simulink library "Control_Library_Rev2"  (R2020b)
settings: Solver=VariableStepAuto  StartTime=0.0  StopTime=10.0  RelTol=1e-3
values from neighbouring files (symbols this model uses):
  Controller_sampleTime = 0.001    [PLC_setup_Rev1_02Mar21.m]    (also in PLC_setup_Rev3.m; PLC_setup_Rev4.m)
  Droop_scaling = 0    [PLC_setup_Rev1_02Mar21.m]    (also in PLC_setup_Rev3.m; PLC_setup_Rev4.m)
  VFD_Adapt_factor_lower_p1458 = 1    [PLC_setup_Rev1_02Mar21.m]    (also in PLC_setup_Rev3.m; PLC_setup_Rev4.m)
  VFD_Adapt_factor_upper_p1459 = 1    [PLC_setup_Rev1_02Mar21.m]    (also in PLC_setup_Rev3.m; PLC_setup_Rev4.m)
  VFD_Curr_limit_var_p0641 = 1    [PLC_setup_Rev1_02Mar21.m]    (also in PLC_setup_Rev3.m; PLC_setup_Rev4.m)
  VFD_Current_limit_p0640 = 430    [PLC_setup_Rev1_02Mar21.m]    (also in PLC_setup_Rev3.m; PLC_setup_Rev4.m)
  VFD_Id_setp_total_r1624 = 73    [PLC_setup_Rev1_02Mar21.m]    (also in PLC_setup_Rev3.m; PLC_setup_Rev4.m)
  VFD_Iq = 1    [PLC_setup_Rev1_02Mar21.m]    (also in PLC_setup_Rev3.m; PLC_setup_Rev4.m)
  VFD_Kp_n_basic_p1460 = 20.174    [PLC_setup_Rev1_02Mar21.m]    (also in PLC_setup_Rev3.m; PLC_setup_Rev4.m)
  VFD_M = inf    [PLC_setup_Rev1_02Mar21.m]    (also in PLC_setup_Rev3.m; PLC_setup_Rev4.m)
  VFD_M_accel_T_smooth_p1517 = 4    [PLC_setup_Rev1_02Mar21.m]    (also in PLC_setup_Rev3.m; PLC_setup_Rev4.m)
  VFD_M_lim_var_fixS_src_p1551 = 1    [PLC_setup_Rev1_02Mar21.m]    (also in PLC_setup_Rev3.m; PLC_setup_Rev4.m)
  VFD_M_max_lower_p1521 = -1345    [PLC_setup_Rev1_02Mar21.m]    (also in PLC_setup_Rev3.m; PLC_setup_Rev4.m)
  VFD_M_max_lower_scal_p1525 = 1    [PLC_setup_Rev1_02Mar21.m]    (also in PLC_setup_Rev3.m; PLC_setup_Rev4.m)
  VFD_M_max_up_mot_scal_p1524 = 1    [PLC_setup_Rev1_02Mar21.m]    (also in PLC_setup_Rev3.m; PLC_setup_Rev4.m)
  VFD_M_max_upper_p1520 = 1345    [PLC_setup_Rev1_02Mar21.m]    (also in PLC_setup_Rev3.m; PLC_setup_Rev4.m)
  VFD_n_act_T_smooth_p1442 = 4    [PLC_setup_Rev1_02Mar21.m]    (also in PLC_setup_Rev3.m; PLC_setup_Rev4.m)
  VFD_n_ctr_Kp_n_up_scal_p1461 = 1    [PLC_setup_Rev1_02Mar21.m]    (also in PLC_setup_Rev3.m; PLC_setup_Rev4.m)
  VFD_n_ctr_Tn_n_up_sca_p1463 = 1    [PLC_setup_Rev1_02Mar21.m]    (also in PLC_setup_Rev3.m; PLC_setup_Rev4.m)
  VFD_n_ctrl_adapt_Kp_lower_p1456 = 0    [PLC_setup_Rev1_02Mar21.m]    (also in PLC_setup_Rev3.m; PLC_setup_Rev4.m)
  VFD_n_ctrl_adapt_Kp_upper_p1457 = 0.1    [PLC_setup_Rev1_02Mar21.m]    (also in PLC_setup_Rev3.m; PLC_setup_Rev4.m)
  VFD_n_ctrl_Adpt_sig_Kp_p1455 = 0    [PLC_setup_Rev1_02Mar21.m]    (also in PLC_setup_Rev3.m; PLC_setup_Rev4.m)
  VFD_n_ctrl_Kp_scal_p1466 = 1    [PLC_setup_Rev1_02Mar21.m]    (also in PLC_setup_Rev3.m; PLC_setup_Rev4.m)
  VFD_n_ctrl_n_lower_p1464 = 0    [PLC_setup_Rev1_02Mar21.m]    (also in PLC_setup_Rev3.m; PLC_setup_Rev4.m)
  VFD_n_ctrl_n_upper_p1465 = 1680    [PLC_setup_Rev1_02Mar21.m]    (also in PLC_setup_Rev3.m; PLC_setup_Rev4.m)
  VFD_n_ctrl_Tn_n_lower_p1462 = 96    [PLC_setup_Rev1_02Mar21.m]    (also in PLC_setup_Rev3.m; PLC_setup_Rev4.m)
  VFD_n_limit_neg_p1086 = -40000    [PLC_setup_Rev1_02Mar21.m]    (also in PLC_setup_Rev3.m; PLC_setup_Rev4.m)
  VFD_n_limit_pos_p1083 = 40000    [PLC_setup_Rev1_02Mar21.m]    (also in PLC_setup_Rev3.m; PLC_setup_Rev4.m)
  VFD_n_limit_setp_p1063 = 40000    [PLC_setup_Rev1_02Mar21.m]    (also in PLC_setup_Rev3.m; PLC_setup_Rev4.m)
  VFD_n_max_p1082 = 1680    [PLC_setup_Rev1_02Mar21.m]    (also in PLC_setup_Rev3.m; PLC_setup_Rev4.m)
  VFD_n_set_filt_1_T_p1416 = 0    [PLC_setup_Rev1_02Mar21.m]    (also in PLC_setup_Rev3.m; PLC_setup_Rev4.m)
  VFD_P_max_gen_p1531 = -375    [PLC_setup_Rev1_02Mar21.m]    (also in PLC_setup_Rev3.m; PLC_setup_Rev4.m)
  VFD_P_max_mot_p1530 = 125    [PLC_setup_Rev1_02Mar21.m]    (also in PLC_setup_Rev3.m; PLC_setup_Rev4.m)
  VFD_PU_I_outp_max_r0289 = 452    [PLC_setup_Rev1_02Mar21.m]    (also in PLC_setup_Rev3.m; PLC_setup_Rev4.m)
  VFD_RFG_ramp_down_time_p1121 = 0.7    [PLC_setup_Rev1_02Mar21.m]    (also in PLC_setup_Rev3.m; PLC_setup_Rev4.m)
  VFD_RFG_ramp_up_time_p1120 = 0.7    [PLC_setup_Rev1_02Mar21.m]    (also in PLC_setup_Rev3.m; PLC_setup_Rev4.m)
  VFD_RFG_t_RD_scal_p1139 = 1    [PLC_setup_Rev1_02Mar21.m]    (also in PLC_setup_Rev3.m; PLC_setup_Rev4.m)
  VFD_RFG_t_RU_scal_p1138 = 1    [PLC_setup_Rev1_02Mar21.m]    (also in PLC_setup_Rev3.m; PLC_setup_Rev4.m)
undefined symbols (not defined in the file or in its folder): DiscIntNeverNeededParam
libraries: simulink x24, $bdroot x2
settings Model: Creator=JillMacPherson  LastModifiedBy=JillMacPherson

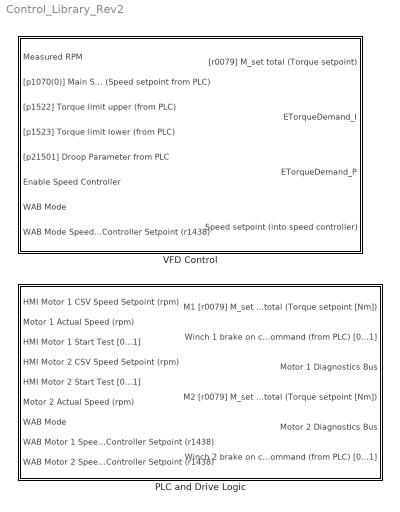
== system Control_Library_Rev2 ==
  PLC and Drive Logic : Subsystem
  VFD Control : Subsystem  TreatAsAtomicUnit=on  SystemSampleTime=Controller_sampleTime

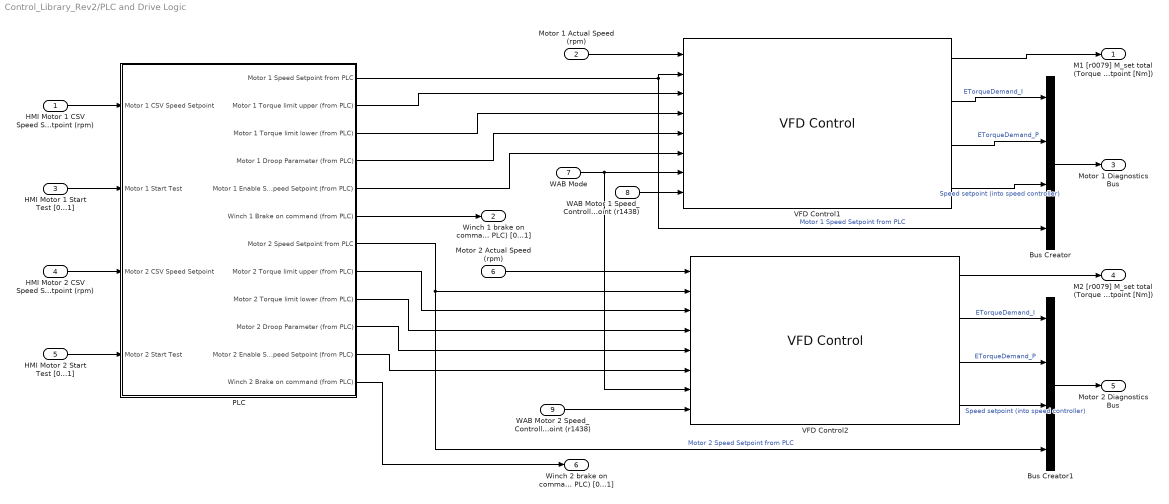
== system Control_Library_Rev2/PLC and Drive Logic ==
  HMI Motor 1 CSV Speed Setpoint (rpm) : Inport
  Motor 1 Actual Speed (rpm) : Inport  Port=2
  HMI Motor 1 Start Test [0...1] : Inport  Port=3
  HMI Motor 2 CSV Speed Setpoint (rpm) : Inport  Port=4
  HMI Motor 2 Start Test [0...1] : Inport  Port=5
  Motor 2 Actual Speed (rpm) : Inport  Port=6
  WAB Mode : Inport  Port=7
  WAB Motor 1 Speed_Controller Setpoint (r1438) : Inport  Port=8
  WAB Motor 2 Speed_Controller Setpoint (r1438) : Inport  Port=9
  Bus Creator : BusCreator  Inputs=4
  Bus Creator1 : BusCreator  Inputs=4
  PLC : Subsystem  TreatAsAtomicUnit=on  SystemSampleTime=Controller_sampleTime
  VFD Control1 : $bdroot/VFD Control  SystemSampleTime=Controller_sampleTime  VariantActivationTime=update diagram  Latency=0  AutoFrameSizeCalculation=off
  VFD Control2 : $bdroot/VFD Control  SystemSampleTime=Controller_sampleTime  VariantActivationTime=update diagram  Latency=0  AutoFrameSizeCalculation=off
  M1 [r0079] M_set total (Torque setpoint [Nm]) : Outport
  Winch 1 brake on command (from PLC) [0...1] : Outport  Port=2
  Motor 1 Diagnostics Bus : Outport  Port=3
  M2 [r0079] M_set total (Torque setpoint [Nm]) : Outport  Port=4
  Motor 2 Diagnostics Bus : Outport  Port=5
  Winch 2 brake on command (from PLC) [0...1] : Outport  Port=6
  wires:
  WAB Motor 2 Speed_Controller Setpoint (r1438)/1 -> VFD Control2/8
  WAB Mode/1 -> VFD Control1/7, VFD Control2/7
  WAB Motor 1 Speed_Controller Setpoint (r1438)/1 -> VFD Control1/8
  PLC/12(Winch 2 Brake on command (from PLC)) -> Winch 2 brake on command (from PLC) [0...1]/1
  PLC/11(Motor 2 Enable Speed Setpoint (from PLC)) -> VFD Control2/6
  PLC/10(Motor 2 Droop Parameter (from PLC)) -> VFD Control2/5
  PLC/9(Motor 2 Torque limit lower (from PLC)) -> VFD Control2/4
  PLC/8(Motor 2 Torque limit upper (from PLC)) -> VFD Control2/3
  PLC/7(Motor 2 Speed Setpoint from PLC) -> VFD Control2/2, Bus Creator1/4  "Motor 2 Speed Setpoint from PLC"
  Motor 2 Actual Speed (rpm)/1 -> VFD Control2/1
  HMI Motor 2 Start Test [0...1]/1 -> PLC/4(Motor 2 Start Test)
  HMI Motor 2 CSV Speed Setpoint (rpm)/1 -> PLC/3(Motor 2 CSV Speed Setpoint)
  PLC/6(Winch 1 Brake on command (from PLC)) -> Winch 1 brake on command (from PLC) [0...1]/1
  VFD Control2/1 -> M2 [r0079] M_set total (Torque setpoint [Nm])/1
  VFD Control2/2 -> Bus Creator1/1  "ETorqueDemand_I"
  VFD Control2/3 -> Bus Creator1/2  "ETorqueDemand_P"
  VFD Control2/4 -> Bus Creator1/3  "Speed setpoint (into speed controller)"
  Bus Creator1/1 -> Motor 2 Diagnostics Bus/1
  Bus Creator/1 -> Motor 1 Diagnostics Bus/1
  VFD Control1/4 -> Bus Creator/3  "Speed setpoint (into speed controller)"
  VFD Control1/3 -> Bus Creator/2  "ETorqueDemand_P"
  VFD Control1/2 -> Bus Creator/1  "ETorqueDemand_I"
  PLC/5(Motor 1 Enable Speed Setpoint (from PLC)) -> VFD Control1/6
  PLC/4(Motor 1 Droop Parameter (from PLC)) -> VFD Control1/5
  HMI Motor 1 CSV Speed Setpoint (rpm)/1 -> PLC/1(Motor 1 CSV Speed Setpoint)
  VFD Control1/1 -> M1 [r0079] M_set total (Torque setpoint [Nm])/1
  HMI Motor 1 Start Test [0...1]/1 -> PLC/2(Motor 1 Start Test)
  PLC/1(Motor 1 Speed Setpoint from PLC) -> Bus Creator/4, VFD Control1/2  "Motor 1 Speed Setpoint from PLC"
  PLC/2(Motor 1 Torque limit upper (from PLC)) -> VFD Control1/3
  Motor 1 Actual Speed (rpm)/1 -> VFD Control1/1
  PLC/3(Motor 1 Torque limit lower (from PLC)) -> VFD Control1/4

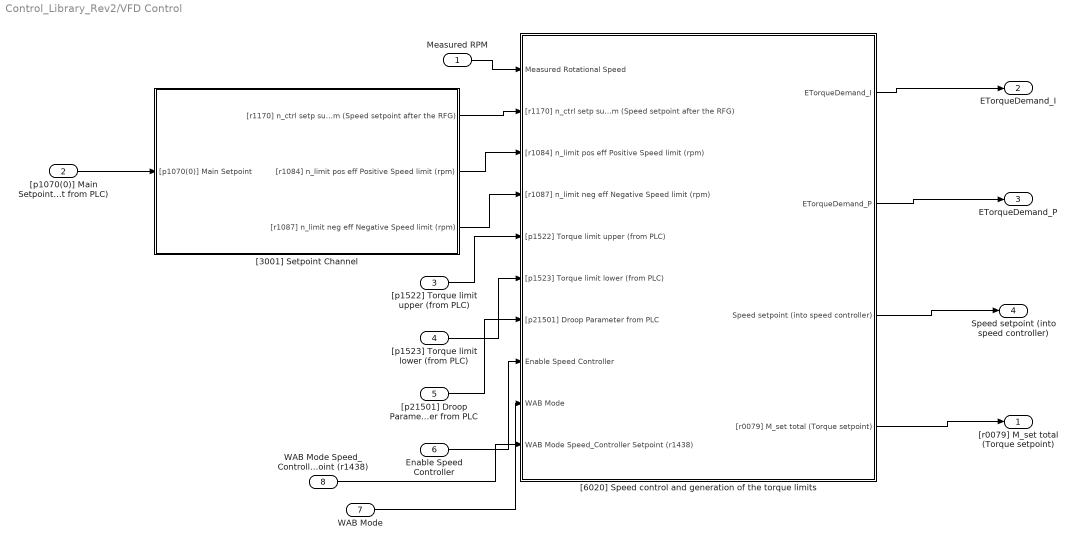
== system Control_Library_Rev2/VFD Control ==
  Measured RPM : Inport
  "[p1070(0)] Main Setpoint (Speed setpoint from PLC)" : Inport  Port=2
  "[p1522] Torque limit upper (from PLC)" : Inport  Port=3
  "[p1523] Torque limit lower (from PLC)" : Inport  Port=4
  "[p21501] Droop Parameter from PLC" : Inport  Port=5
  Enable Speed Controller : Inport  Port=6
  WAB Mode : Inport  Port=7
  WAB Mode Speed_Controller Setpoint (r1438) : Inport  Port=8
  "[3001] Setpoint Channel " : Subsystem
  "[6020] Speed control and generation of the torque limits " : Subsystem
  "[r0079] M_set total (Torque setpoint)" : Outport  VectorParamsAs1DForOutWhenUnconnected=off
  ETorqueDemand_I : Outport  Port=2  VectorParamsAs1DForOutWhenUnconnected=off
  ETorqueDemand_P : Outport  Port=3  VectorParamsAs1DForOutWhenUnconnected=off
  Speed setpoint (into speed controller) : Outport  Port=4  VectorParamsAs1DForOutWhenUnconnected=off
  wires:
  WAB Mode Speed_Controller Setpoint (r1438)/1 -> "[6020] Speed control and generation of the torque limits "/10(WAB Mode Speed_Controller Setpoint (r1438))
  WAB Mode/1 -> "[6020] Speed control and generation of the torque limits "/9(WAB Mode)
  "[6020] Speed control and generation of the torque limits "/1(ETorqueDemand_I) -> ETorqueDemand_I/1
  "[6020] Speed control and generation of the torque limits "/2(ETorqueDemand_P) -> ETorqueDemand_P/1
  Measured RPM/1 -> "[6020] Speed control and generation of the torque limits "/1(Measured Rotational Speed)
  "[p1070(0)] Main Setpoint (Speed setpoint from PLC)"/1 -> "[3001] Setpoint Channel "/1("[p1070(0)] Main Setpoint")
  "[3001] Setpoint Channel "/1("[r1170] n_ctrl setp sum (Speed setpoint after the RFG)") -> "[6020] Speed control and generation of the torque limits "/2("[r1170] n_ctrl setp sum (Speed setpoint after the RFG)")
  "[3001] Setpoint Channel "/2("[r1084] n_limit pos eff Positive Speed limit (rpm)") -> "[6020] Speed control and generation of the torque limits "/3("[r1084] n_limit pos eff Positive Speed limit (rpm)")
  "[3001] Setpoint Channel "/3("[r1087] n_limit neg eff Negative Speed limit (rpm)") -> "[6020] Speed control and generation of the torque limits "/4("[r1087] n_limit neg eff Negative Speed limit (rpm)")
  "[6020] Speed control and generation of the torque limits "/3(Speed setpoint (into speed controller)) -> Speed setpoint (into speed controller)/1
  "[6020] Speed control and generation of the torque limits "/4("[r0079] M_set total (Torque setpoint)") -> "[r0079] M_set total (Torque setpoint)"/1
  "[p1523] Torque limit lower (from PLC)"/1 -> "[6020] Speed control and generation of the torque limits "/6("[p1523] Torque limit lower (from PLC)")
  "[p1522] Torque limit upper (from PLC)"/1 -> "[6020] Speed control and generation of the torque limits "/5("[p1522] Torque limit upper (from PLC)")
  "[p21501] Droop Parameter from PLC"/1 -> "[6020] Speed control and generation of the torque limits "/7("[p21501] Droop Parameter from PLC")
  Enable Speed Controller/1 -> "[6020] Speed control and generation of the torque limits "/8(Enable Speed Controller)

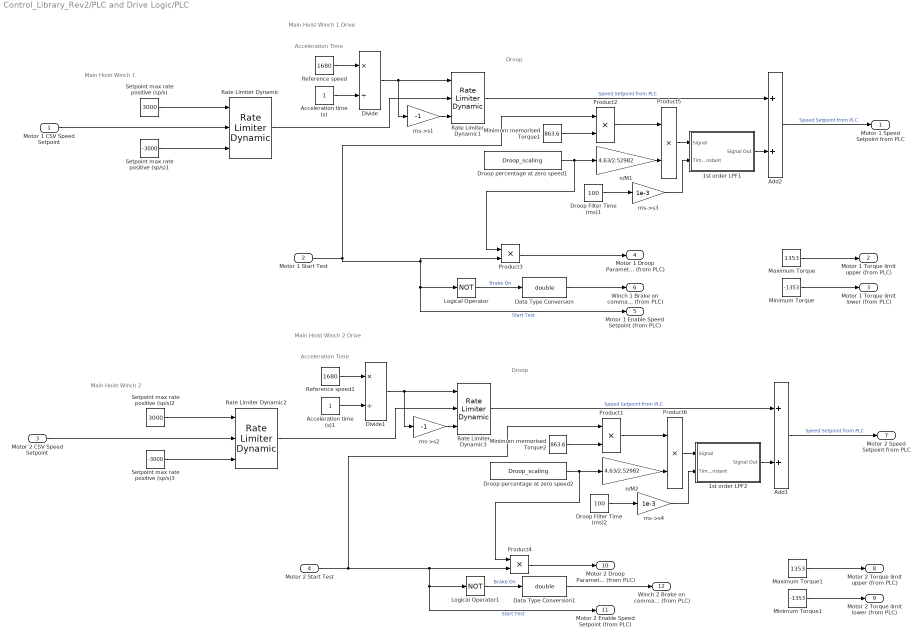
== system Control_Library_Rev2/PLC and Drive Logic/PLC ==
  note: Main Hoist Winch 2
  note: Droop
  note: Acceleration Time
  note: Main Hoist Winch 2 Drive
  note: Main Hoist Winch 1
  note: Droop
  note: Acceleration Time
  note: Main Hoist Winch 1 Drive
  Motor 1 CSV Speed Setpoint : Inport
  Motor 1 Start Test : Inport  Port=2
  Motor 2 CSV Speed Setpoint : Inport  Port=3
  Motor 2 Start Test : Inport  Port=4
  1st order LPF1 : Subsystem  mask{time_constant=0.1, Yo=0}
      mask prompts: time_constant "Time Constant (s)"; Yo "Initial Condition"
  1st order LPF2 : Subsystem  mask{time_constant=0.1, Yo=0}
      mask prompts: time_constant "Time Constant (s)"; Yo "Initial Condition"
  Acceleration time (s) : Constant
  Acceleration time (s)1 : Constant
  Add1 : Sum
  Add2 : Sum
  Data Type Conversion : DataTypeConversion  OutDataTypeStr=double
  Data Type Conversion1 : DataTypeConversion  OutDataTypeStr=double
  Divide : Product  Inputs=*/
  Divide1 : Product  Inputs=*/
  Droop Filter Time (ms)1 : Constant  Value=100
  Droop Filter Time (ms)2 : Constant  Value=100
  Droop percentage at zero speed1 : Constant  Value=Droop_scaling
  Droop percentage at zero speed2 : Constant  Value=Droop_scaling
  Logical Operator : Logic  Operator=NOT  AllPortsSameDT=off  OutDataTypeStr=boolean
  Logical Operator1 : Logic  Operator=NOT  AllPortsSameDT=off  OutDataTypeStr=boolean
  Maximum Torque : Constant  Value=1353
  Maximum Torque1 : Constant  Value=1353
  Minimum Torque : Constant  Value=-1353
  Minimum Torque1 : Constant  Value=-1353
  Minimum memorised Torque1 : Constant  Value=863.6
  Minimum memorised Torque2 : Constant  Value=863.6
  Product{1..2,5..6} (4 alike) : Product  Inputs=**
  Product3 : Product
  Product4 : Product
  Rate Limiter Dynamic{,1..3} (4 alike) : simulink/Discontinuities/Rate Limiter Dynamic
  Reference speed : Constant  Value=1680
  Reference speed1 : Constant  Value=1680
  Setpoint max rate positive (sp/s) : Constant  Value=3000
  Setpoint max rate positive (sp/s)1 : Constant  Value=-3000
  Setpoint max rate positive (sp/s)2 : Constant  Value=3000
  Setpoint max rate positive (sp/s)3 : Constant  Value=-3000
  ms->s1 : Gain  Gain=-1
  ms->s2 : Gain  Gain=-1
  ms->s3 : Gain  Gain=1e-3
  ms->s4 : Gain  Gain=1e-3
  n/M1 : Gain  Gain=4.63/2.52982
  n/M2 : Gain  Gain=4.63/2.52982
  Motor 1 Speed Setpoint from PLC : Outport
  Motor 1 Torque limit upper (from PLC) : Outport  Port=2
  Motor 1 Torque limit lower (from PLC) : Outport  Port=3
  Motor 1 Droop Parameter (from PLC) : Outport  Port=4
  Motor 1 Enable Speed Setpoint (from PLC) : Outport  Port=5
  Winch 1 Brake on command (from PLC) : Outport  Port=6
  Motor 2 Speed Setpoint from PLC : Outport  Port=7
  Motor 2 Torque limit upper (from PLC) : Outport  Port=8
  Motor 2 Torque limit lower (from PLC) : Outport  Port=9
  Motor 2 Droop Parameter (from PLC) : Outport  Port=10
  Motor 2 Enable Speed Setpoint (from PLC) : Outport  Port=11
  Winch 2 Brake on command (from PLC) : Outport  Port=12
  wires:
  Product1/1 -> Product6/1
  n/M2/1 -> Product6/2
  ms->s2/1 -> Rate Limiter Dynamic3/3
  ms->s4/1 -> 1st order LPF2/2(Time Constant)
  Divide1/1 -> ms->s2/1, Rate Limiter Dynamic3/1
  Setpoint max rate positive (sp/s)2/1 -> Rate Limiter Dynamic2/1
  Setpoint max rate positive (sp/s)3/1 -> Rate Limiter Dynamic2/3
  Product6/1 -> 1st order LPF2/1(Signal)
  Droop Filter Time (ms)2/1 -> ms->s4/1
  1st order LPF2/1(Signal Out) -> Add1/2
  Droop percentage at zero speed2/1 -> Product4/1, n/M2/1
  Rate Limiter Dynamic2/1 -> Rate Limiter Dynamic3/2
  Minimum memorised Torque2/1 -> Product1/2
  Reference speed1/1 -> Divide1/1
  Acceleration time (s)1/1 -> Divide1/2
  Add1/1 -> Motor 2 Speed Setpoint from PLC/1  "Speed Setpoint from PLC"
  Maximum Torque1/1 -> Motor 2 Torque limit upper (from PLC)/1
  Minimum Torque1/1 -> Motor 2 Torque limit lower (from PLC)/1
  Rate Limiter Dynamic3/1 -> Add1/1  "Speed Setpoint from PLC"
  Motor 2 Start Test/1 -> Product4/2, Logical Operator1/1, Motor 2 Enable Speed Setpoint (from PLC)/1, Product1/1  "Start Test"
  Product4/1 -> Motor 2 Droop Parameter (from PLC)/1
  Logical Operator1/1 -> Data Type Conversion1/1  "Brake On"
  Data Type Conversion1/1 -> Winch 2 Brake on command (from PLC)/1
  Motor 2 CSV Speed Setpoint/1 -> Rate Limiter Dynamic2/2
  Motor 1 CSV Speed Setpoint/1 -> Rate Limiter Dynamic/2
  Data Type Conversion/1 -> Winch 1 Brake on command (from PLC)/1
  Logical Operator/1 -> Data Type Conversion/1  "Brake On"
  Product3/1 -> Motor 1 Droop Parameter (from PLC)/1
  Motor 1 Start Test/1 -> Product2/1, Product3/2, Logical Operator/1, Motor 1 Enable Speed Setpoint (from PLC)/1  "Start Test"
  Rate Limiter Dynamic1/1 -> Add2/1  "Speed Setpoint from PLC"
  Minimum Torque/1 -> Motor 1 Torque limit lower (from PLC)/1
  Maximum Torque/1 -> Motor 1 Torque limit upper (from PLC)/1
  Add2/1 -> Motor 1 Speed Setpoint from PLC/1  "Speed Setpoint from PLC"
  Acceleration time (s)/1 -> Divide/2
  Reference speed/1 -> Divide/1
  Minimum memorised Torque1/1 -> Product2/2
  Rate Limiter Dynamic/1 -> Rate Limiter Dynamic1/2
  Droop percentage at zero speed1/1 -> n/M1/1, Product3/1
  1st order LPF1/1(Signal Out) -> Add2/2
  Droop Filter Time (ms)1/1 -> ms->s3/1
  Product5/1 -> 1st order LPF1/1(Signal)
  Setpoint max rate positive (sp/s)1/1 -> Rate Limiter Dynamic/3
  Setpoint max rate positive (sp/s)/1 -> Rate Limiter Dynamic/1
  Divide/1 -> Rate Limiter Dynamic1/1, ms->s1/1
  ms->s3/1 -> 1st order LPF1/2(Time Constant)
  ms->s1/1 -> Rate Limiter Dynamic1/3
  n/M1/1 -> Product5/2
  Product2/1 -> Product5/1

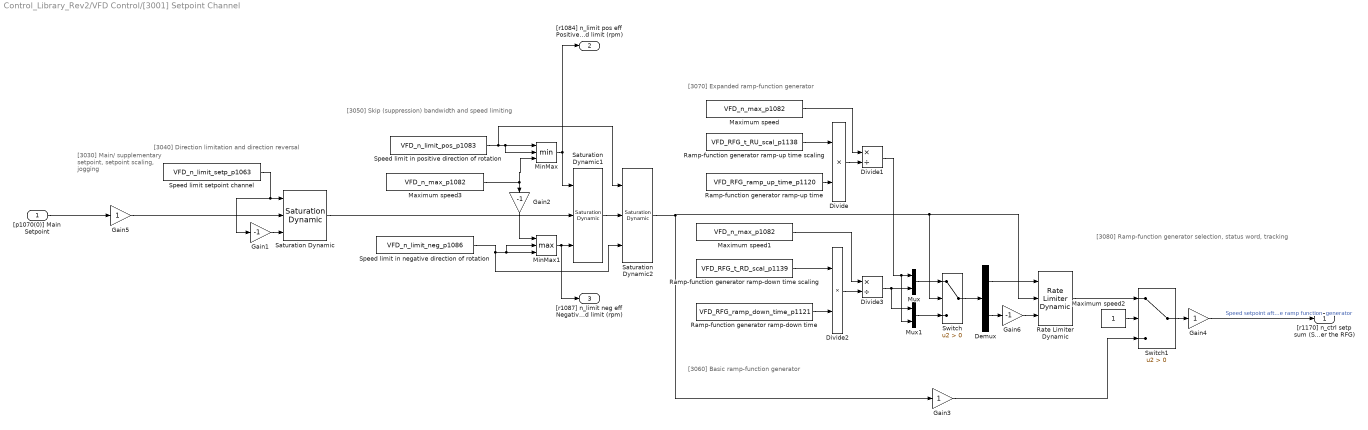
== system Control_Library_Rev2/VFD Control/[3001] Setpoint Channel  ==
  note: [3080] Ramp-function generator selection,
      | status word, tracking
  note: [3070] Expanded ramp-function generator
  note: [3040] Direction limitation and direction reversal
  note: [3050] Skip (suppression) bandwidth
      |  and speed limiting
  note: [3060] Basic ramp-function generator
  note: [3030] Main/
      | supplementary
      | setpoint,
      | setpoint
      | scaling,
      | jogging
  "[p1070(0)] Main Setpoint" : Inport
  Demux : Demux  Outputs=2
  Divide : Product  Inputs=**
  Divide1 : Product  Inputs=*/
  Divide2 : Product  Inputs=**
  Divide3 : Product  Inputs=*/
  Gain1 : Gain  Gain=-1
  Gain2 : Gain  Gain=-1
  Gain3 : Gain
  Gain4 : Gain
  Gain5 : Gain
  Gain6 : Gain  Gain=-1
  Maximum speed : Constant  Value=VFD_n_max_p1082
  Maximum speed1 : Constant  Value=VFD_n_max_p1082
  Maximum speed2 : Constant
  Maximum speed3 : Constant  Value=VFD_n_max_p1082
  MinMax : MinMax  Inputs=3
  MinMax1 : MinMax  Function=max  Inputs=3
  Mux : Mux  Inputs=2
  Mux1 : Mux  Inputs=2
  Ramp-function generator ramp-down time : Constant  Value=VFD_RFG_ramp_down_time_p1121
  Ramp-function generator ramp-down time scaling : Constant  Value=VFD_RFG_t_RD_scal_p1139  VectorParams1D=off
  "Ramp-function generator ramp-up time " : Constant  Value=VFD_RFG_ramp_up_time_p1120
  "Ramp-function generator ramp-up time scaling " : Constant  Value=VFD_RFG_t_RU_scal_p1138
  Rate Limiter Dynamic : simulink/Discontinuities/Rate Limiter Dynamic
  Saturation Dynamic : simulink/Discontinuities/Saturation Dynamic  OutMin=[]  OutMax=[]  OutDataTypeStr=Inherit: Same as second input  OutDataType=fixdt(1, 16)  OutScaling=2^-10  DoSatur=off
  Saturation Dynamic1 : simulink/Discontinuities/Saturation Dynamic  OutMin=[]  OutMax=[]  OutDataTypeStr=Inherit: Same as second input  OutDataType=fixdt(1, 16)  OutScaling=2^-10  DoSatur=off
  Saturation Dynamic2 : simulink/Discontinuities/Saturation Dynamic  OutMin=[]  OutMax=[]  OutDataTypeStr=Inherit: Same as second input  OutDataType=fixdt(1, 16)  OutScaling=2^-10  DoSatur=off
  "Speed limit in negative direction of rotation " : Constant  Value=VFD_n_limit_neg_p1086
  Speed limit in positive direction of rotation : Constant  Value=VFD_n_limit_pos_p1083
  Speed limit setpoint channel : Constant  Value=VFD_n_limit_setp_p1063
  Switch : Switch  Criteria=u2 > Threshold
  Switch1 : Switch  Criteria=u2 > Threshold
  "[r1170] n_ctrl setp sum (Speed setpoint after the RFG)" : Outport  VectorParamsAs1DForOutWhenUnconnected=off
  "[r1084] n_limit pos eff Positive Speed limit (rpm)" : Outport  Port=2  VectorParamsAs1DForOutWhenUnconnected=off
  "[r1087] n_limit neg eff Negative Speed limit (rpm)" : Outport  Port=3  VectorParamsAs1DForOutWhenUnconnected=off
  wires:
  Speed limit setpoint channel/1 -> Saturation Dynamic/1, Gain1/1
  Gain1/1 -> Saturation Dynamic/3
  "[p1070(0)] Main Setpoint"/1 -> Gain5/1
  MinMax1/1 -> "[r1087] n_limit neg eff Negative Speed limit (rpm)"/1, Saturation Dynamic1/3
  Saturation Dynamic/1 -> Saturation Dynamic1/2
  Speed limit in positive direction of rotation/1 -> Saturation Dynamic2/1, MinMax/2, MinMax/1
  "Speed limit in negative direction of rotation "/1 -> Saturation Dynamic2/3, MinMax1/2, MinMax1/3
  Maximum speed3/1 -> Gain2/1, MinMax/3
  MinMax/1 -> "[r1084] n_limit pos eff Positive Speed limit (rpm)"/1, Saturation Dynamic1/1
  Saturation Dynamic2/1 -> Gain3/1, Rate Limiter Dynamic/2, Switch/2
  Mux/1 -> Switch/1
  Maximum speed/1 -> Divide1/1
  Demux/2 -> Gain6/1
  Divide3/1 -> Mux1/1, Mux/2
  "Ramp-function generator ramp-up time scaling "/1 -> Divide/1
  Mux1/1 -> Switch/3
  Switch/1 -> Demux/1
  Divide1/1 -> Mux/1, Mux1/2
  "Ramp-function generator ramp-up time "/1 -> Divide/2
  Divide2/1 -> Divide3/2
  Maximum speed1/1 -> Divide3/1
  Ramp-function generator ramp-down time scaling/1 -> Divide2/1
  Ramp-function generator ramp-down time/1 -> Divide2/2
  Divide/1 -> Divide1/2
  Demux/1 -> Rate Limiter Dynamic/1
  Gain4/1 -> "[r1170] n_ctrl setp sum (Speed setpoint after the RFG)"/1  "Speed setpoint after  the ramp function  generator"
  Rate Limiter Dynamic/1 -> Switch1/1
  Switch1/1 -> Gain4/1
  Gain3/1 -> Switch1/3
  Maximum speed2/1 -> Switch1/2
  Gain5/1 -> Saturation Dynamic/2
  Gain6/1 -> Rate Limiter Dynamic/3
  Saturation Dynamic1/1 -> Saturation Dynamic2/2
  Gain2/1 -> MinMax1/1

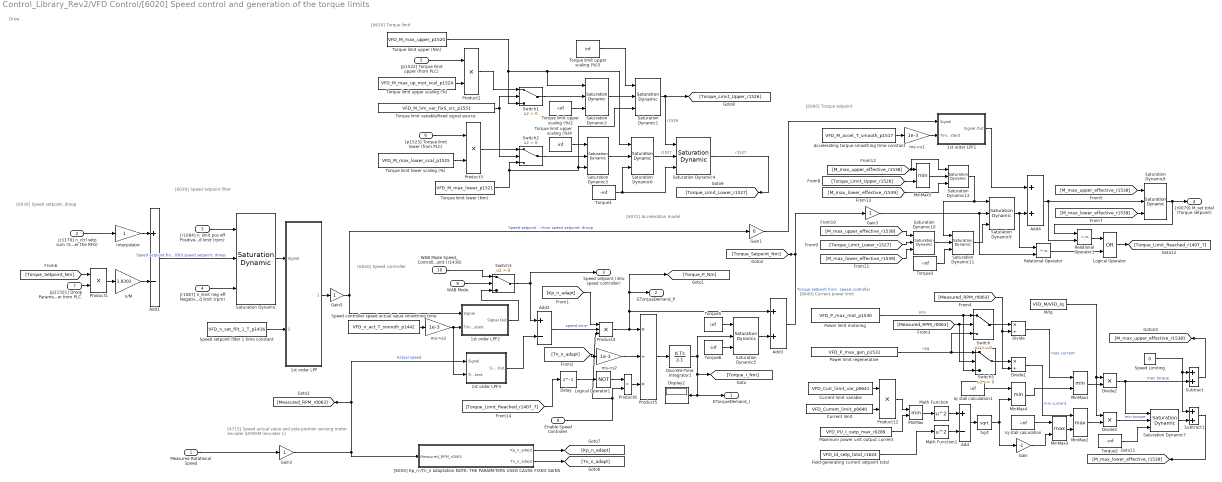
== system Control_Library_Rev2/VFD Control/[6020] Speed control and generation of the torque limits  ==
  note: [6030] Speed setpoint filter
  note: [6031] Acceleration model
  note: [4715] Speed actual value and pole position
      |  sensing motor encoder ASM/SM (encoder 1)
  note: [6630] Torque limit
  note: Drive
  note: [6030] Speed setpoint, droop
  note: [6040] Speed controller
  note: [6060] Torque setpoint
  note: [6640] Current-power limit
  Measured Rotational Speed : Inport
  "[r1170] n_ctrl setp sum (Speed setpoint after the RFG)" : Inport  Port=2
  "[r1084] n_limit pos eff Positive Speed limit (rpm)" : Inport  Port=3
  "[r1087] n_limit neg eff Negative Speed limit (rpm)" : Inport  Port=4
  "[p1522] Torque limit upper (from PLC)" : Inport  Port=5
  "[p1523] Torque limit lower (from PLC)" : Inport  Port=6
  "[p21501] Droop Parameter from PLC" : Inport  Port=7
  Enable Speed Controller : Inport  Port=8
  WAB Mode : Inport  Port=9
  WAB Mode Speed_Controller Setpoint (r1438) : Inport  Port=10
  1st order LPF : Subsystem  mask{time_constant=0.1, Yo=0}
      mask prompts: time_constant "Time Constant (s)"; Yo "Initial Condition"
  1st order LPF1 : Subsystem  mask{time_constant=0.1, Yo=0}
      mask prompts: time_constant "Time Constant (s)"; Yo "Initial Condition"
  1st order LPF2 : Subsystem  mask{time_constant=0.1, Yo=0}
      mask prompts: time_constant "Time Constant (s)"; Yo "Initial Condition"
  1st order LPF3 : Subsystem  mask{time_constant=0.1, Yo=0}
      mask prompts: time_constant "Time Constant (s)"; Yo "Initial Condition"
  Accelerating torque smoothing time constant : Constant  Value=VFD_M_accel_T_smooth_p1517
  Add : Sum  Inputs=+-
  Add1 : Sum  Inputs=+-
  Add2 : Sum  Inputs=+-
  Add3 : Sum
  Add4 : Sum
  Current limit : Constant  Value=VFD_Current_limit_p0640
  Current limit variable : Constant  Value=VFD_Curr_limit_var_p0641
  Delay : Delay  DelayLength=1
  Discrete-Time Integrator1 : DiscreteIntegrator  SampleTime=0.001  ICPrevOutput=DiscIntNeverNeededParam  ICPrevScaledInput=DiscIntNeverNeededParam
  Display2 : Display
  Divide : Product  Inputs=*/
  Divide1 : Product  Inputs=*/
  Divide2 : Product  Inputs=**
  Divide3 : Product  Inputs=**
  Field-generating current setpoint total : Constant  Value=VFD_Id_setp_total_r1624
  Gain : Gain  Gain=-1
  Gain1 : Gain  Gain=0
  Gain2 : Gain
  Gain3 : Gain
  Gain5 : Gain
  Interpolator : Gain
  Iq stall calculation : Constant  Value=-inf
  Iq stall calculation1 : Constant  Value=inf
  Logical Operator : Logic  Operator=OR  AllPortsSameDT=off  OutDataTypeStr=boolean
  Logical Operator1 : Logic  Operator=NOT  AllPortsSameDT=off  OutDataTypeStr=boolean
  M/Iq : Constant  Value=VFD_M/VFD_Iq
  Math Function : Math  Operator=square  SaturateOnIntegerOverflow=on
  Math Function1 : Math  Operator=square  SaturateOnIntegerOverflow=on
  Maximum power unit output current : Constant  Value=VFD_PU_I_outp_max_r0289
  MinMax{,1,4..5} (4 alike) : MinMax  Inputs=2
  MinMax2 : MinMax  Function=max  Inputs=2
  MinMax3 : MinMax  Function=max  Inputs=2
  Power limit motoring : Constant  Value=VFD_P_max_mot_p1530
  Power limit regenerative : Constant  Value=VFD_P_max_gen_p1531
  Product1 : Product  Inputs=**
  Product12 : Product
  Product2 : Product
  Product3 : Product
  Product4 : Product  Inputs=3
  Product5 : Product  Inputs=*/*
  Product6 : Product  Inputs=**
  Relational Operator : RelationalOperator  Operator=~=  OutDataTypeStr=boolean  RndMeth=Simplest
  Relational Operator1 : RelationalOperator  Operator=~=  OutDataTypeStr=boolean  RndMeth=Simplest
  Saturation Dynamic{,1..12} (13 alike) : simulink/Discontinuities/Saturation Dynamic  OutMin=[]  OutMax=[]  OutDataTypeStr=Inherit: Same as second input  OutDataType=fixdt(1, 16)  OutScaling=2^-10  DoSatur=off
  Speed Limiting : Constant  Value=0
  Speed controller speed actual value smoothing time : Constant  Value=VFD_n_act_T_smooth_p1442
  "Speed setpoint filter 1 time constant " : Constant  Value=VFD_n_set_filt_1_T_p1416
  Sqrt : Sqrt  SaturateOnIntegerOverflow=on
  Subtract : Sum
  Subtract1 : Sum
  Switch : Switch
  Switch1 : Switch  Criteria=u2 > Threshold
  Switch2 : Switch  Criteria=u2 > Threshold
  Switch3 : Switch  Criteria=u2 > Threshold
  Switch5 : Switch
  Torque limit lower (Nm) : Constant  Value=VFD_M_max_lower_p1521
  Torque limit lower scaling (%) : Constant  Value=VFD_M_max_lower_scal_p1525
  Torque limit upper (Nm) : Constant  Value=VFD_M_max_upper_p1520
  Torque limit upper scaling (%) : Constant  Value=VFD_M_max_up_mot_scal_p1524
  Torque limit upper scaling (%)2 : Constant  Value=-inf
  Torque limit upper scaling (%)3 : Constant  Value=inf
  Torque limit upper scaling (%)4 : Constant  Value=inf
  Torque limit variable/fixed signal source : Constant  Value=VFD_M_lim_var_fixS_src_p1551
  Torque{1..3,6} (4 alike) : Constant  Value=-inf
  Torque5 : Constant  Value=inf
  "[6050] Kp_n-/Tn_n adaptation NOTE: THE PARAMETERS USED CAUSE FIXED GAINS" : Subsystem
  ms->s1 : Gain  Gain=1e-3
  ms->s2 : Gain  Gain=1e-3
  ms->s3 : Gain  Gain=1e-3
  n/M : Gain  Gain=1.8302
  ETorqueDemand_I : Outport  VectorParamsAs1DForOutWhenUnconnected=off
  ETorqueDemand_P : Outport  Port=2  VectorParamsAs1DForOutWhenUnconnected=off
  Speed setpoint (into speed controller) : Outport  Port=3  VectorParamsAs1DForOutWhenUnconnected=off
  "[r0079] M_set total (Torque setpoint)" : Outport  Port=4  VectorParamsAs1DForOutWhenUnconnected=off
  wires:
  WAB Mode Speed_Controller Setpoint (r1438)/1 -> Switch3/1
  1st order LPF2/1(Signal Out) -> Switch3/3
  WAB Mode/1 -> Switch3/2
  Measured Rotational Speed/1 -> Gain2/1
  Saturation Dynamic/1 -> 1st order LPF/1(Signal)
  "[r1084] n_limit pos eff Positive Speed limit (rpm)"/1 -> Saturation Dynamic/1
  "[r1087] n_limit neg eff Negative Speed limit (rpm)"/1 -> Saturation Dynamic/3
  "Speed setpoint filter 1 time constant "/1 -> 1st order LPF/2(Time Constant)
  Product2/1 -> Switch1/1
  Switch1/1 -> Saturation Dynamic2/2
  Switch2/1 -> Saturation Dynamic3/2
  Saturation Dynamic3/1 -> Saturation Dynamic6/2
  Saturation Dynamic1/1 -> [Torque_Limit_Upper_r1526], Saturation Dynamic4/1  "r1526"
  Torque1/1 -> Saturation Dynamic4/3, Saturation Dynamic6/3
  Torque limit upper (Nm)/1 -> Switch1/3, Saturation Dynamic6/1, Saturation Dynamic2/1
  "[p1522] Torque limit upper (from PLC)"/1 -> Product2/1
  Torque limit upper scaling (%)/1 -> Product2/2
  Torque limit lower (Nm)/1 -> Switch2/3, Saturation Dynamic3/3, Saturation Dynamic1/3
  Torque limit lower scaling (%)/1 -> Product3/2
  Saturation Dynamic4/1 -> [Torque_Limit_Lower_r1527]  "r1527"
  [Torque_Setpoint_Nm] -> Product1/1
  Discrete-Time Integrator1/1 -> [Torque_I_Nm], ETorqueDemand_I/1, Display2/1, Saturation Dynamic5/2
  Switch3/1 -> Speed setpoint (into speed controller)/1, Add2/1
  Product1/1 -> n/M/1
  [Tn_n_adapt] -> ms->s2/1
  Saturation Dynamic5/1 -> Add3/2
  Interpolator/1 -> Add1/1
  Product4/1 -> Product5/1, Add3/1, ETorqueDemand_P/1, [Torque_P_Nm]
  n/M/1 -> Add1/2
  [Kp_n_adapt] -> Product4/1
  Torque6/1 -> Saturation Dynamic5/3
  Add2/1 -> Product4/2  "speed error"
  Torque5/1 -> Saturation Dynamic5/1
  Add3/1 -> [Torque_Setpoint_Nm], Gain3/1  "Torque setpoint from  speed controller"
  Product5/1 -> Discrete-Time Integrator1/1
  ms->s2/1 -> Product5/2
  1st order LPF/1(Signal Out) -> Gain5/1
  Speed controller speed actual value smoothing time/1 -> ms->s3/1
  Gain5/1 -> Gain1/1, 1st order LPF2/1(Signal)  "Speed setpoint from speed setpoint, droop"
  Gain2/1 -> "[6050] Kp_n-/Tn_n adaptation NOTE: THE PARAMETERS USED CAUSE FIXED GAINS"/1(Measured_RPM_r0063), [Measured_RPM_r0063], 1st order LPF3/1(Signal)  "Actual speed"
  ms->s3/1 -> 1st order LPF2/2(Time Constant), 1st order LPF3/2(Time Constant)
  1st order LPF3/1(Signal Out) -> Add2/2
  Saturation Dynamic8/1 -> Relational Operator1/1, "[r0079] M_set total (Torque setpoint)"/1
  Torque limit variable/fixed signal source/1 -> Switch1/2, Switch2/2
  Torque limit upper scaling (%)2/1 -> Saturation Dynamic2/3
  Saturation Dynamic2/1 -> Saturation Dynamic1/2
  Torque limit upper scaling (%)3/1 -> Saturation Dynamic1/1
  "[p1523] Torque limit lower (from PLC)"/1 -> Product3/1
  Product3/1 -> Switch2/1
  Torque limit upper scaling (%)4/1 -> Saturation Dynamic3/1
  Saturation Dynamic6/1 -> Saturation Dynamic4/2  "r1527"
  Power limit regenerative/1 -> Switch5/1, Switch/3  "neg"
  Power limit motoring/1 -> Switch5/3, Switch/1  "pos"
  [Measured_RPM_r0063] -> Switch5/2, Switch/2
  Switch/1 -> Divide/1
  Switch5/1 -> Divide1/1
  [Measured_RPM_r0063] -> Divide1/2, Divide/2
  Current limit variable/1 -> Product12/1
  Current limit/1 -> Product12/2
  Product12/1 -> MinMax/1
  Maximum power unit output current/1 -> MinMax/2
  MinMax/1 -> Math Function/1
  Field-generating current setpoint total/1 -> Math Function1/1
  Math Function/1 -> Add/1
  Math Function1/1 -> Add/2
  Add/1 -> Sqrt/1
  Sqrt/1 -> MinMax4/2, Gain/1
  Divide/1 -> MinMax1/1  "max current"
  Divide1/1 -> MinMax2/1  "min current"
  Gain/1 -> MinMax3/2
  MinMax1/1 -> Divide2/2
  MinMax2/1 -> Divide3/2
  M/Iq/1 -> Divide2/1, Divide3/1
  Divide3/1 -> Saturation Dynamic7/2  "min torque"
  Torque2/1 -> Saturation Dynamic7/3
  Divide2/1 -> Subtract/2, Saturation Dynamic7/1  "max torque"
  Speed Limiting/1 -> Subtract/1, Subtract1/1
  Saturation Dynamic7/1 -> Subtract1/2
  Subtract/1 -> [M_max_upper_effective_r1538]
  Subtract1/1 -> [M_max_lower_effective_r1539]
  MinMax3/1 -> MinMax2/2
  Iq stall calculation/1 -> MinMax3/1
  MinMax4/1 -> MinMax1/2
  Iq stall calculation1/1 -> MinMax4/1
  "[6050] Kp_n-/Tn_n adaptation NOTE: THE PARAMETERS USED CAUSE FIXED GAINS"/2(Tn_n_adapt) -> [Tn_n_adapt]
  [M_max_upper_effective_r1538] -> Saturation Dynamic8/1
  [M_max_lower_effective_r1539] -> Saturation Dynamic8/3
  Add4/1 -> Relational Operator1/2, Saturation Dynamic8/2
  1st order LPF1/1(Signal Out) -> Add4/1
  Gain3/1 -> Saturation Dynamic9/2, Relational Operator/2
  Saturation Dynamic9/1 -> Add4/2, Relational Operator/1
  [Torque_Limit_Lower_r1527] -> Saturation Dynamic10/2
  Saturation Dynamic11/1 -> Saturation Dynamic9/3
  [M_max_upper_effective_r1538] -> Saturation Dynamic10/1
  [M_max_lower_effective_r1539] -> Saturation Dynamic10/3
  Torque3/1 -> Saturation Dynamic11/3
  Saturation Dynamic10/1 -> Saturation Dynamic11/2
  [Torque_Limit_Upper_r1526] -> MinMax5/2
  [M_max_upper_effective_r1538] -> Saturation Dynamic12/1, MinMax5/1
  Saturation Dynamic12/1 -> Saturation Dynamic9/1, Saturation Dynamic11/1
  MinMax5/1 -> Saturation Dynamic12/2
  [M_max_lower_effective_r1539] -> Saturation Dynamic12/3
  Relational Operator/1 -> Logical Operator/2
  Relational Operator1/1 -> Logical Operator/1
  Logical Operator/1 -> [Torque_Limit_Reached_r1407_7]
  [Torque_Limit_Reached_r1407_7] -> Delay/1
  Product6/1 -> Product5/3
  Accelerating torque smoothing time constant/1 -> ms->s1/1
  ms->s1/1 -> 1st order LPF1/2(Time Constant)
  Gain1/1 -> 1st order LPF1/1(Signal)
  Delay/1 -> Logical Operator1/1
  Add1/1 -> Saturation Dynamic/2  "Speed setpoint from  [6030] speed setpoint, droop"
  "[r1170] n_ctrl setp sum (Speed setpoint after the RFG)"/1 -> Interpolator/1
  "[6050] Kp_n-/Tn_n adaptation NOTE: THE PARAMETERS USED CAUSE FIXED GAINS"/1(Kp_n_adapt) -> [Kp_n_adapt]
  "[p21501] Droop Parameter from PLC"/1 -> Product1/2
  Logical Operator1/1 -> Product6/1
  Enable Speed Controller/1 -> Product4/3, Product6/2

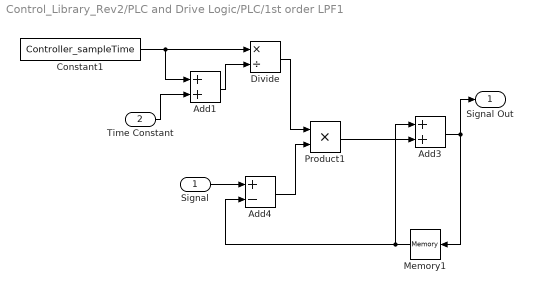
== system Control_Library_Rev2/PLC and Drive Logic/PLC/1st order LPF1 ==
  Signal : Inport
  Time Constant : Inport  Port=2
  Add1 : Sum
  Add3 : Sum
  Add4 : Sum  Inputs=+-
  Constant1 : Constant  Value=Controller_sampleTime
  Divide : Product  Inputs=*/
  Memory1 : Memory  InitialCondition=Yo  InheritSampleTime=on
  Product1 : Product  RndMeth=Zero
  Signal Out : Outport  VectorParamsAs1DForOutWhenUnconnected=off
  wires:
  Signal/1 -> Add4/1
  Constant1/1 -> Divide/1, Add1/1
  Time Constant/1 -> Add1/2
  Add4/1 -> Product1/2
  Memory1/1 -> Add3/1, Add4/2
  Product1/1 -> Add3/2
  Add3/1 -> Signal Out/1, Memory1/1
  Divide/1 -> Product1/1
  Add1/1 -> Divide/2

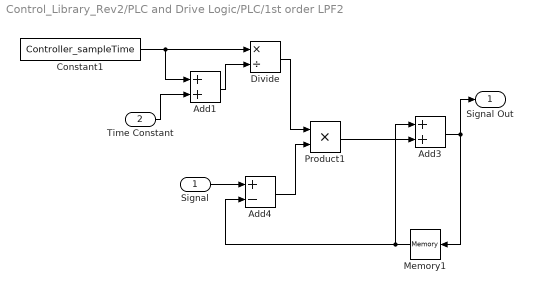
== system Control_Library_Rev2/PLC and Drive Logic/PLC/1st order LPF2 ==
  Signal : Inport
  Time Constant : Inport  Port=2
  Add1 : Sum
  Add3 : Sum
  Add4 : Sum  Inputs=+-
  Constant1 : Constant  Value=Controller_sampleTime
  Divide : Product  Inputs=*/
  Memory1 : Memory  InitialCondition=Yo  InheritSampleTime=on
  Product1 : Product  RndMeth=Zero
  Signal Out : Outport  VectorParamsAs1DForOutWhenUnconnected=off
  wires:
  Add1/1 -> Divide/2
  Divide/1 -> Product1/1
  Add3/1 -> Memory1/1, Signal Out/1
  Product1/1 -> Add3/2
  Memory1/1 -> Add4/2, Add3/1
  Add4/1 -> Product1/2
  Time Constant/1 -> Add1/2
  Constant1/1 -> Add1/1, Divide/1
  Signal/1 -> Add4/1

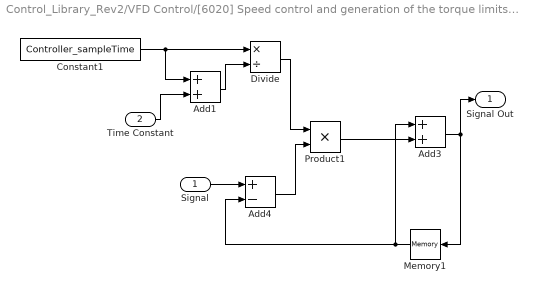
== system Control_Library_Rev2/VFD Control/[6020] Speed control and generation of the torque limits /1st order LPF ==
  Signal : Inport
  Time Constant : Inport  Port=2
  Add1 : Sum
  Add3 : Sum
  Add4 : Sum  Inputs=+-
  Constant1 : Constant  Value=Controller_sampleTime
  Divide : Product  Inputs=*/
  Memory1 : Memory  InitialCondition=Yo  InheritSampleTime=on
  Product1 : Product  RndMeth=Zero
  Signal Out : Outport  VectorParamsAs1DForOutWhenUnconnected=off
  wires:
  Signal/1 -> Add4/1
  Constant1/1 -> Divide/1, Add1/1
  Time Constant/1 -> Add1/2
  Add4/1 -> Product1/2
  Memory1/1 -> Add3/1, Add4/2
  Product1/1 -> Add3/2
  Add3/1 -> Signal Out/1, Memory1/1
  Divide/1 -> Product1/1
  Add1/1 -> Divide/2

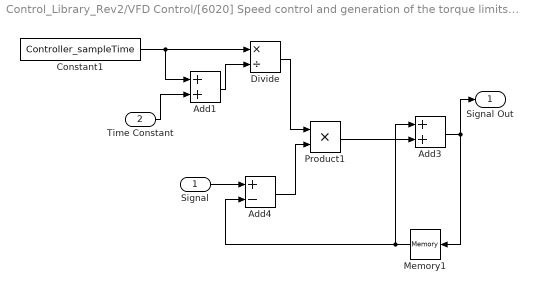
== system Control_Library_Rev2/VFD Control/[6020] Speed control and generation of the torque limits /1st order LPF1 ==
  Signal : Inport
  Time Constant : Inport  Port=2
  Add1 : Sum
  Add3 : Sum
  Add4 : Sum  Inputs=+-
  Constant1 : Constant  Value=Controller_sampleTime
  Divide : Product  Inputs=*/
  Memory1 : Memory  InitialCondition=Yo  InheritSampleTime=on
  Product1 : Product  RndMeth=Zero
  Signal Out : Outport  VectorParamsAs1DForOutWhenUnconnected=off
  wires:
  Signal/1 -> Add4/1
  Constant1/1 -> Divide/1, Add1/1
  Time Constant/1 -> Add1/2
  Add4/1 -> Product1/2
  Memory1/1 -> Add3/1, Add4/2
  Product1/1 -> Add3/2
  Add3/1 -> Signal Out/1, Memory1/1
  Divide/1 -> Product1/1
  Add1/1 -> Divide/2

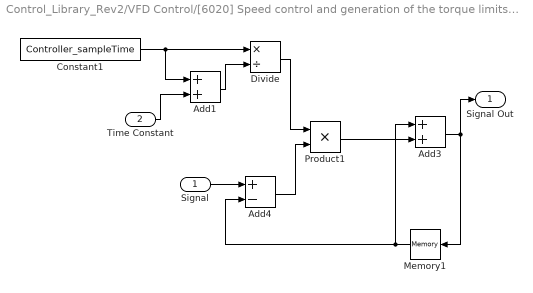
== system Control_Library_Rev2/VFD Control/[6020] Speed control and generation of the torque limits /1st order LPF2 ==
  Signal : Inport
  Time Constant : Inport  Port=2
  Add1 : Sum
  Add3 : Sum
  Add4 : Sum  Inputs=+-
  Constant1 : Constant  Value=Controller_sampleTime
  Divide : Product  Inputs=*/
  Memory1 : Memory  InitialCondition=Yo  InheritSampleTime=on
  Product1 : Product  RndMeth=Zero
  Signal Out : Outport  VectorParamsAs1DForOutWhenUnconnected=off
  wires:
  Add1/1 -> Divide/2
  Divide/1 -> Product1/1
  Add3/1 -> Memory1/1, Signal Out/1
  Product1/1 -> Add3/2
  Memory1/1 -> Add4/2, Add3/1
  Add4/1 -> Product1/2
  Time Constant/1 -> Add1/2
  Constant1/1 -> Add1/1, Divide/1
  Signal/1 -> Add4/1

== system Control_Library_Rev2/VFD Control/[6020] Speed control and generation of the torque limits /1st order LPF3 ==
  Signal : Inport
  Time Constant : Inport  Port=2
  Add1 : Sum
  Add3 : Sum
  Add4 : Sum  Inputs=+-
  Constant1 : Constant  Value=Controller_sampleTime
  Divide : Product  Inputs=*/
  Memory1 : Memory  InitialCondition=Yo  InheritSampleTime=on
  Product1 : Product  RndMeth=Zero
  Signal Out : Outport  VectorParamsAs1DForOutWhenUnconnected=off
  wires:
  Signal/1 -> Add4/1
  Constant1/1 -> Divide/1, Add1/1
  Time Constant/1 -> Add1/2
  Add4/1 -> Product1/2
  Memory1/1 -> Add3/1, Add4/2
  Product1/1 -> Add3/2
  Add3/1 -> Signal Out/1, Memory1/1
  Divide/1 -> Product1/1
  Add1/1 -> Divide/2

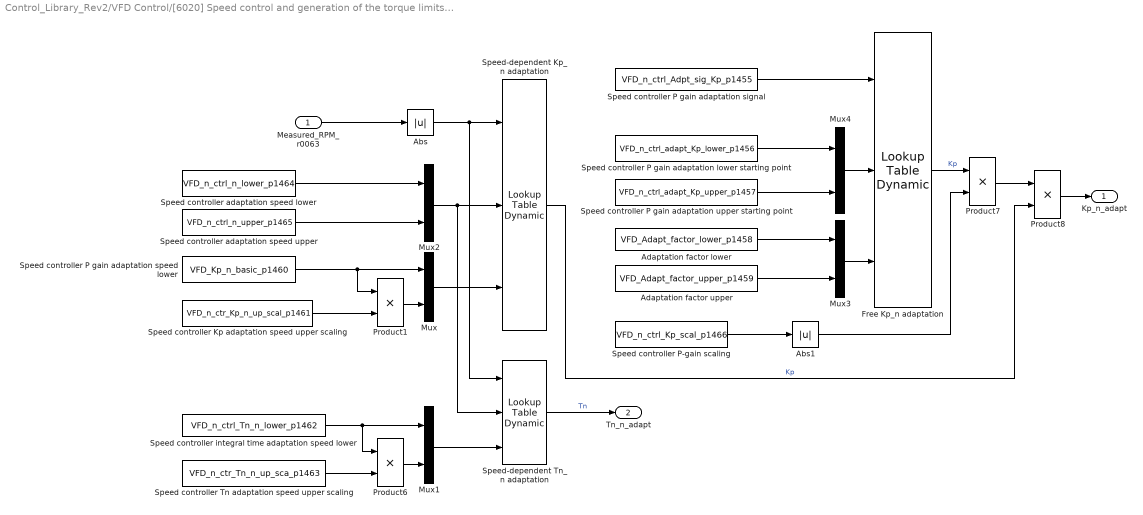
== system Control_Library_Rev2/VFD Control/[6020] Speed control and generation of the torque limits /[6050] Kp_n-//Tn_n adaptation NOTE: THE PARAMETERS USED CAUSE FIXED GAINS ==
  Measured_RPM_r0063 : Inport
  Abs : Abs
  Abs1 : Abs
  Adaptation factor lower : Constant  Value=VFD_Adapt_factor_lower_p1458
  "Adaptation factor upper " : Constant  Value=VFD_Adapt_factor_upper_p1459
  Free Kp_n adaptation : simulink/Lookup Tables/Lookup Table Dynamic  LookUpMeth=Interpolation-Use End Values  OutDataType=fixdt('double')  OutScaling=[]  OutputDataTypeScalingMode=Specify via dialog  OutDataTypeStr=double  DoSatur=off
  Mux{,1..4} (5 alike) : Mux  Inputs=2
  Product{1,6..8} (4 alike) : Product  Inputs=**
  Speed controller Kp adaptation speed upper scaling : Constant  Value=VFD_n_ctr_Kp_n_up_scal_p1461
  Speed controller P gain adaptation lower starting point : Constant  Value=VFD_n_ctrl_adapt_Kp_lower_p1456
  "Speed controller P gain adaptation signal " : Constant  Value=VFD_n_ctrl_Adpt_sig_Kp_p1455
  Speed controller P gain adaptation speed lower : Constant  Value=VFD_Kp_n_basic_p1460
  Speed controller P gain adaptation upper starting point : Constant  Value=VFD_n_ctrl_adapt_Kp_upper_p1457
  Speed controller P-gain scaling : Constant  Value=VFD_n_ctrl_Kp_scal_p1466
  Speed controller Tn adaptation speed upper scaling : Constant  Value=VFD_n_ctr_Tn_n_up_sca_p1463
  "Speed controller adaptation speed lower " : Constant  Value=VFD_n_ctrl_n_lower_p1464
  Speed controller adaptation speed upper : Constant  Value=VFD_n_ctrl_n_upper_p1465
  Speed controller integral time adaptation speed lower : Constant  Value=VFD_n_ctrl_Tn_n_lower_p1462
  Speed-dependent Kp_n adaptation : simulink/Lookup Tables/Lookup Table Dynamic  LookUpMeth=Interpolation-Use End Values  OutDataType=fixdt('double')  OutScaling=[]  OutputDataTypeScalingMode=Specify via dialog  OutDataTypeStr=double  DoSatur=off
  Speed-dependent Tn_n adaptation : simulink/Lookup Tables/Lookup Table Dynamic  LookUpMeth=Interpolation-Use End Values  OutDataType=fixdt('double')  OutScaling=[]  OutputDataTypeScalingMode=Specify via dialog  OutDataTypeStr=double  DoSatur=off
  Kp_n_adapt : Outport
  Tn_n_adapt : Outport  Port=2
  wires:
  Product1/1 -> Mux/2
  Abs/1 -> Speed-dependent Kp_n adaptation/1, Speed-dependent Tn_n adaptation/1
  Abs1/1 -> Product7/2
  Adaptation factor lower/1 -> Mux3/1
  "Speed controller adaptation speed lower "/1 -> Mux2/1
  "Speed controller P gain adaptation signal "/1 -> Free Kp_n adaptation/1
  Speed controller integral time adaptation speed lower/1 -> Mux1/1, Product6/1
  Speed-dependent Tn_n adaptation/1 -> Tn_n_adapt/1  "Tn"
  Speed controller P gain adaptation speed lower/1 -> Product1/1, Mux/1
  Speed-dependent Kp_n adaptation/1 -> Product8/2  "Kp"
  Speed controller Tn adaptation speed upper scaling/1 -> Product6/2
  Mux1/1 -> Speed-dependent Tn_n adaptation/3
  Mux2/1 -> Speed-dependent Kp_n adaptation/2, Speed-dependent Tn_n adaptation/2
  Product7/1 -> Product8/1
  Product6/1 -> Mux1/2
  Speed controller adaptation speed upper/1 -> Mux2/2
  Speed controller P-gain scaling/1 -> Abs1/1
  Speed controller Kp adaptation speed upper scaling/1 -> Product1/2
  Measured_RPM_r0063/1 -> Abs/1
  Free Kp_n adaptation/1 -> Product7/1  "Kp"
  Mux/1 -> Speed-dependent Kp_n adaptation/3
  Speed controller P gain adaptation lower starting point/1 -> Mux4/1
  Speed controller P gain adaptation upper starting point/1 -> Mux4/2
  Mux3/1 -> Free Kp_n adaptation/3
  "Adaptation factor upper "/1 -> Mux3/2
  Mux4/1 -> Free Kp_n adaptation/2
  Product8/1 -> Kp_n_adapt/1
